simulink model "SLIP_simulink"  (R2017a)
settings: Solver=VariableStepAuto  StartTime=0.0  StopTime=10  RelTol=1e-3
model workspace (MAT data in the model file):
  k = Simulink.Parameter
  k.Value = 20000
  k.DataType = 'auto'
  k.Dimensions = [1 1]
  l_0 = Simulink.Parameter
  l_0.Value = 1
  l_0.DataType = 'auto'
  l_0.Dimensions = [1 1]
  m = Simulink.Parameter
  m.Value = 80
  m.DataType = 'auto'
  m.Dimensions = [1 1]
  touchdown_angle = Simulink.Parameter
  touchdown_angle.Value = 1.57079632679
  touchdown_angle.DataType = 'auto'
  touchdown_angle.Dimensions = [1 1]
values from neighbouring files (symbols this model uses):
  k = parameter.k    [BSLIP.m]    (also in SLIP.m = 100; SLIP3D.m; SLIP_m.m = 100; test.m = 100)
  m = parameter.m    [BSLIP.m]    (also in SLIP.m = 1; SLIP3D.m; SLIP_m.m = 1; test.m = 1)
  touchdown_angle = pi/180 * 77.8    (= 1.35786615805)    [SLIP.m]    (also in SLIP_m.m = 1.57079632679; test.m = 1.57079632679)
settings Model: Creator=steffen  LastModifiedBy=steffen

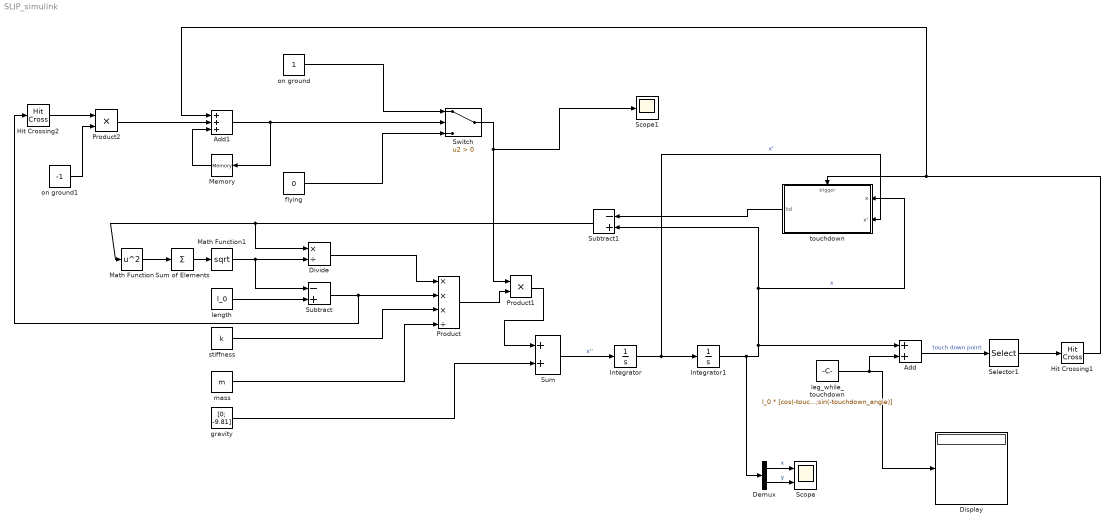
== system SLIP_simulink ==
  Add : Sum
  Add1 : Sum  Inputs=+++
  Demux : Demux  Outputs=2
  Display : Display
  Divide : Product  Inputs=*/  OutDataTypeStr=double
  Hit Crossing1 : HitCross  HitCrossingDirection=falling
  Hit Crossing2 : HitCross  HitCrossingDirection=falling
  Integrator : Integrator  InitialCondition=[1.3;0]
  Integrator1 : Integrator  InitialCondition=[1;2]
  Math Function : Math  Operator=square  SaturateOnIntegerOverflow=on
  Math Function1 : Math  Operator=sqrt  SaturateOnIntegerOverflow=on
  Memory : Memory
  Product : Product  Inputs=***/
  Product1 : Product
  Product2 : Product
  Scope : Scope  NumInputPorts=2
  Scope1 : Scope
  Selector1 : Selector  InputPortWidth=2  IndexOptions=Index vector (dialog)  Indices=[2]  OutputSizes=1
  Subtract : Sum  Inputs=-+
  Subtract1 : Sum  Inputs=-+
  Sum : Sum
  Sum of Elements : Sum  Inputs=+
  Switch : Switch  Criteria=u2 > Threshold
  flying : Constant  Value=0
  gravity : Constant  Value=[0; -9.81]  VectorParams1D=off
  leg_while_touchdown : Constant  Value=l_0 * [cos(-touchdown_angle);sin(-touchdown_angle)]  VectorParams1D=off
  length : Constant  Value=l_0
  mass : Constant  Value=m
  on ground : Constant
  on ground1 : Constant  Value=-1
  stiffness : Constant  Value=k
  touchdown : Subsystem
  wires:
  Integrator/1 -> touchdown/2(x'), Integrator1/1  "x'"
  Integrator1/1 -> Demux/1, touchdown/1(x), Subtract1/2, Add/1  "x"
  Sum/1 -> Integrator/1  "x''"
  stiffness/1 -> Product/3
  length/1 -> Subtract/2
  Subtract1/1 -> Math Function/1, Divide/1
  Sum of Elements/1 -> Math Function1/1
  Math Function/1 -> Sum of Elements/1
  Math Function1/1 -> Subtract/1, Divide/2
  Divide/1 -> Product/1
  Subtract/1 -> Hit Crossing2/1, Product/2
  mass/1 -> Product/4
  gravity/1 -> Sum/2
  Product/1 -> Product1/2
  touchdown/1(td) -> Subtract1/1
  Hit Crossing1/1 -> Add1/1, touchdown/Trigger
  Demux/1 -> Scope/1  "x"
  Demux/2 -> Scope/2  "y"
  leg_while_touchdown/1 -> Display/1, Add/2
  Add/1 -> Selector1/1  "touch down point"
  Selector1/1 -> Hit Crossing1/1
  flying/1 -> Switch/3
  on ground/1 -> Switch/1
  Product1/1 -> Sum/1
  Switch/1 -> Scope1/1, Product1/1
  Add1/1 -> Memory/1, Switch/2
  Memory/1 -> Add1/3
  Product2/1 -> Add1/2
  Hit Crossing2/1 -> Product2/1
  on ground1/1 -> Product2/2

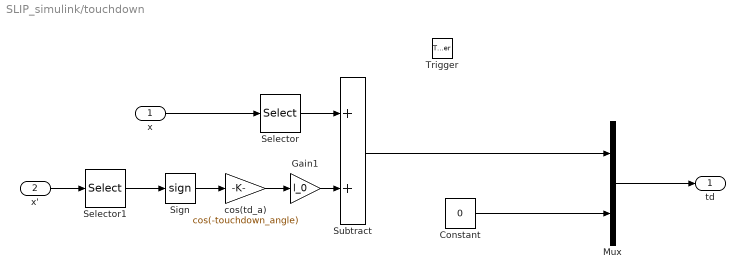
== system SLIP_simulink/touchdown ==
  x : Inport
  x' : Inport  Port=2
  Trigger : TriggerPort  VariantControl=Variant  PortDimensions=1
  Constant : Constant  Value=0
  Gain1 : Gain  Gain=l_0
  Mux : Mux  Inputs=2
  Selector : Selector  InputPortWidth=2  IndexOptions=Index vector (dialog)  Indices=[1]  OutputSizes=1
  Selector1 : Selector  InputPortWidth=2  IndexOptions=Index vector (dialog)  Indices=[1]  OutputSizes=1
  Sign : Signum
  Subtract : Sum
  cos(td_a) : Gain  Gain=cos(-touchdown_angle)
  td : Outport
  wires:
  x/1 -> Selector/1
  Selector/1 -> Subtract/1
  Constant/1 -> Mux/2
  Subtract/1 -> Mux/1
  x'/1 -> Selector1/1
  Selector1/1 -> Sign/1
  Sign/1 -> cos(td_a)/1
  Gain1/1 -> Subtract/2
  cos(td_a)/1 -> Gain1/1
  Mux/1 -> td/1
